simulink model "HW3_P4"  (R2017a)
settings: Solver=VariableStepAuto  StartTime=0.0  StopTime=10.0  RelTol=1e-3
settings Model: Creator=Merc  LastModifiedBy=Merc

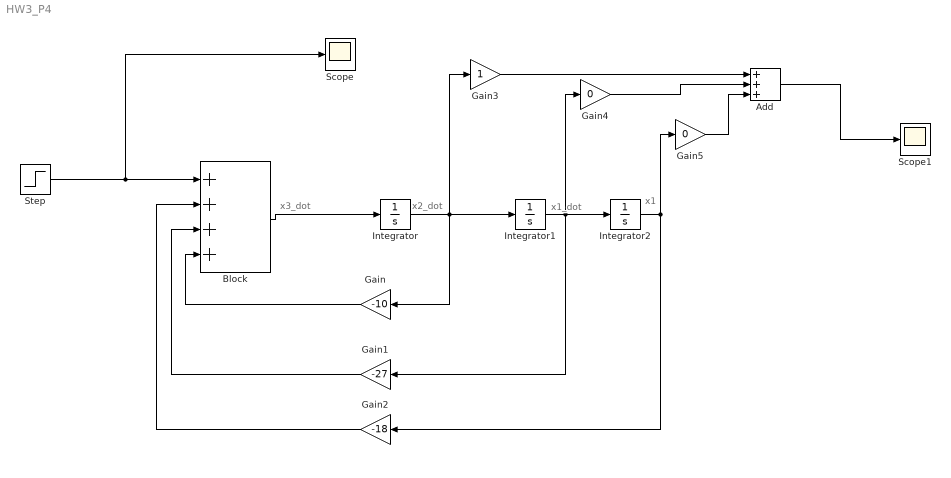
== system HW3_P4 ==
  note: x1
  note: x1_dot
  note: x2_dot
  note: x3_dot
  Add : Sum  Inputs=3
  Block : Sum  Inputs=++++
  Gain : Gain  Gain=-10
  Gain1 : Gain  Gain=-27
  Gain2 : Gain  Gain=-18
  Gain3 : Gain
  Gain4 : Gain  Gain=0
  Gain5 : Gain  Gain=0
  Integrator : Integrator
  Integrator1 : Integrator
  Integrator2 : Integrator
  Scope : Scope
  Scope1 : Scope
  Step : Step  SampleTime=1
  wires:
  Block/1 -> Integrator/1
  Integrator/1 -> Gain3/1, Integrator1/1, Gain/1
  Integrator1/1 -> Gain4/1, Integrator2/1, Gain1/1
  Integrator2/1 -> Gain5/1, Gain2/1
  Step/1 -> Scope/1, Block/1
  Gain/1 -> Block/4
  Gain1/1 -> Block/3
  Gain2/1 -> Block/2
  Gain3/1 -> Add/1
  Gain4/1 -> Add/2
  Gain5/1 -> Add/3
  Add/1 -> Scope1/1
